simulink model "gncDeputy"  (R2023a)
settings: Solver=ode4  StartTime=0.0  StopTime=10.0  FixedStep=dt_gnc  RelTol=1e-3
values from neighbouring files (symbols this model uses):
  dv_cmd = zeros(3,3)    [swarmMaitenance.m]
  M_cmd = zeros(1,3)    [swarmMaitenance.m]
undefined symbols (not defined in the file or in its folder): controlWindows, dt_gnc, environment, gnc_override
libraries: aerolibutil x1
settings Model: Creator=ndelurgio  LastModifiedBy=ndelurgio

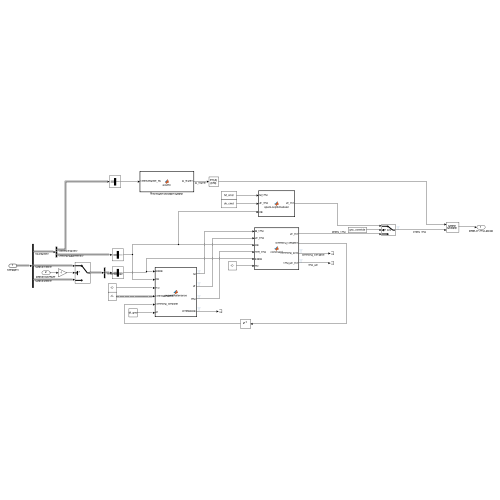
[thumbnail: Simulink's stored preview of the top-level diagram]
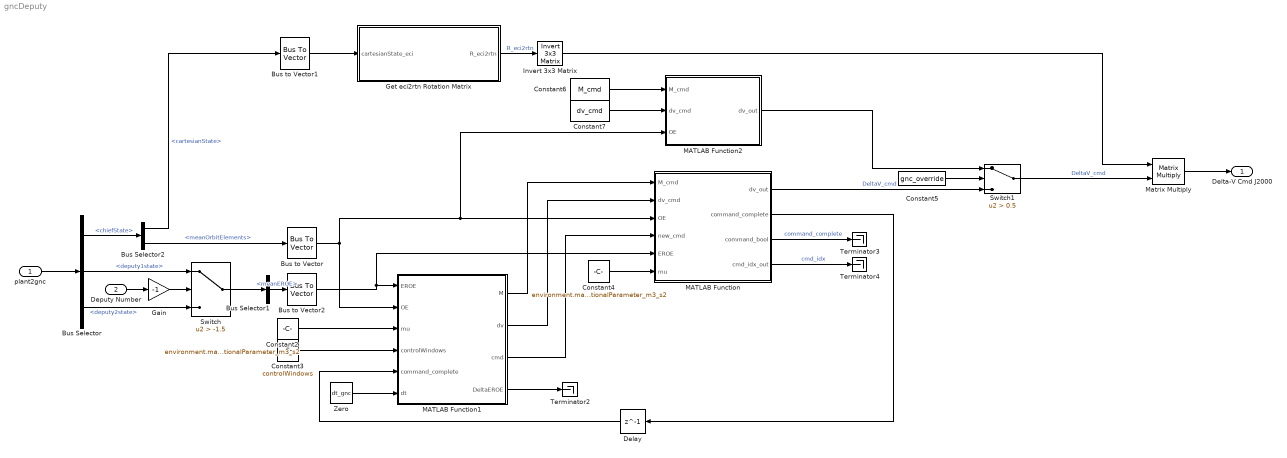
== system gncDeputy ==
  plant2gnc : Inport  OutDataTypeStr=Bus: plant2gnc
  Deputy Number : Inport  Port=2
  Bus Selector : BusSelector  OutputSignals=chiefState,deputy1state,deputy2state
  Bus Selector1 : BusSelector  OutputSignals=meanEROE
  Bus Selector2 : BusSelector  OutputSignals=cartesianState,meanOrbitElements
  Bus to Vector : BusToVector
  Bus to Vector1 : BusToVector
  Bus to Vector2 : BusToVector
  Constant2 : Constant  Value=environment.marsProperties.gravitationalParameter_m3_s2
  Constant3 : Constant  Value=controlWindows  OutDataTypeStr=Bus: controlWindowsBus
  Constant4 : Constant  Value=environment.marsProperties.gravitationalParameter_m3_s2
  Constant5 : Constant  Value=gnc_override
  Constant6 : Constant  Value=M_cmd
  Constant7 : Constant  Value=dv_cmd
  Delay : Delay  DelayLength=1  InitialCondition=false
  Gain : Gain  Gain=-1
  Get eci2rtn Rotation Matrix : MATLAB Function  TreatAsAtomicUnit=on
  Invert 3x3 Matrix : aerolibutil/Invert  3x3 Matrix
  MATLAB Function : MATLAB Function  TreatAsAtomicUnit=on
  MATLAB Function1 : MATLAB Function  TreatAsAtomicUnit=on
  MATLAB Function2 : MATLAB Function  TreatAsAtomicUnit=on
  Matrix Multiply : Product  Multiplication=Matrix(*)
  Switch : Switch  Criteria=u2 > Threshold  Threshold=-1.5  SaturateOnIntegerOverflow=off  InputSameDT=off
  Switch1 : Switch  Criteria=u2 > Threshold  Threshold=0.5  SaturateOnIntegerOverflow=off  InputSameDT=off
  Terminator2 : Terminator
  Terminator3 : Terminator
  Terminator4 : Terminator
  Zero : Constant  Value=dt_gnc  OutDataTypeStr=Inherit: Inherit via back propagation
  Delta-V Cmd J2000 : Outport
  wires:
  MATLAB Function/1(dv_out) -> Switch1/3  "DeltaV_cmd"
  plant2gnc/1 -> Bus Selector/1
  Bus Selector/2 -> Switch/1  "<deputy1state>"
  Bus Selector/3 -> Switch/3  "<deputy2state>"
  Bus Selector/1 -> Bus Selector2/1  "<chiefState>"
  Deputy Number/1 -> Gain/1
  Switch/1 -> Bus Selector1/1
  Bus Selector1/1 -> Bus to Vector2/1  "<meanEROE>"
  Gain/1 -> Switch/2
  Bus Selector2/2 -> Bus to Vector/1  "<meanOrbitElements>"
  Bus Selector2/1 -> Bus to Vector1/1  "<cartesianState>"
  Bus to Vector1/1 -> Get eci2rtn Rotation Matrix/1(cartesianState_eci)
  Get eci2rtn Rotation Matrix/1(R_eci2rtn) -> Invert 3x3 Matrix/1  "R_eci2rtn"
  Invert 3x3 Matrix/1 -> Matrix Multiply/1
  Matrix Multiply/1 -> Delta-V Cmd J2000/1
  MATLAB Function1/3(cmd) -> MATLAB Function/4(new_cmd)
  Bus to Vector2/1 -> MATLAB Function/5(EROE), MATLAB Function1/1(EROE)
  Constant2/1 -> MATLAB Function1/3(mu)
  Constant3/1 -> MATLAB Function1/4(controlWindows)
  MATLAB Function/2(command_complete) -> Delay/1
  Delay/1 -> MATLAB Function1/5(command_complete)
  MATLAB Function1/1(M) -> MATLAB Function/1(M_cmd)
  MATLAB Function1/2(dv) -> MATLAB Function/2(dv_cmd)
  MATLAB Function1/4(DeltaEROE) -> Terminator2/1
  Constant4/1 -> MATLAB Function/6(mu)
  MATLAB Function/3(command_bool) -> Terminator3/1  "command_complete"
  Zero/1 -> MATLAB Function1/6(dt)
  MATLAB Function/4(cmd_idx_out) -> Terminator4/1  "cmd_idx"
  Switch1/1 -> Matrix Multiply/2  "DeltaV_cmd"
  Constant5/1 -> Switch1/2
  MATLAB Function2/1(dv_out) -> Switch1/1
  Constant6/1 -> MATLAB Function2/1(M_cmd)
  Constant7/1 -> MATLAB Function2/2(dv_cmd)
  Bus to Vector/1 -> MATLAB Function1/2(OE), MATLAB Function2/3(OE), MATLAB Function/3(OE)

== matlab function gncDeputy/Get eci2rtn Rotation Matrix ==
  data: cartesianState_eci input; R_eci2rtn output
function R_eci2rtn  = eci2rtn(cartesianState_eci)

[~, R_eci2rtn] = eci2rtn(cartesianState_eci);

end

== matlab function gncDeputy/MATLAB Function ==
  data: M_cmd input size=[3 1]; dv_out output double size=[3 1]; dv_cmd input size=[3 3]; OE input size=[6 1]; new_cmd input size=1; command_complete output boolean size=1; EROE input size=[6 1]; mu input size=1; command_bool output size=1; cmd_idx_out output size=1
function [dv_out, command_complete, command_bool, cmd_idx_out] = command(M_cmd,dv_cmd,OE, new_cmd, EROE, mu)
[dv_out, command_complete, command_bool, cmd_idx_out] = command(M_cmd,dv_cmd,OE, new_cmd, EROE, mu);
end

== matlab function gncDeputy/MATLAB Function1 ==
  data: EROE input; M output; OE input; mu input; controlWindows input; command_complete input boolean; dv output; cmd output; DeltaEROE output; dt input
function [M,dv,cmd,DeltaEROE] = swarmMaitenance(EROE,OE,mu,controlWindows, command_complete, dt)
[M,dv,cmd,DeltaEROE] = swarmMaitenance(EROE,OE,mu,controlWindows, command_complete, dt);
end

== matlab function gncDeputy/MATLAB Function2 ==
  data: M_cmd input; dv_out output; dv_cmd input; OE input
function dv_out = openLoopScheduler(M_cmd,dv_cmd,OE)
dv_out = openLoopScheduler(M_cmd,dv_cmd,OE);
end
